simulink model "hdlcoder_ofdm_fft_eml_1024b"  (R2014a)
settings: Solver=FixedStepDiscrete  SolverMode=SingleTasking  StartTime=0.0  StopTime=35000  RelTol=1e-3
InitFcn:
  | wordLength = 16;
  | fracLength = 10;
  | TotalPoint= 1024;
  | TotalStage= 10;
  | FFT_nt=numerictype(1,12, 6);
  | twiddle_Signed = 1;
  | twiddle_WordLength = 12;
  | twiddle_FractionLength = 10;
  | twiddle_nt=numerictype(1,12, 10);
undefined symbols (not defined in the file): EbNodB, M
libraries: dspxfrm3 x3, commdigbbndpm3 x3, commsink2 x2, commchan3 x1, simulink x1, commrandsrc2 x1
Description:
  | OFDM Receiver with 512-Point Serial FFT
  | This model shows how to use Simulink(R) HDL Coder(TM) to check, generate,
  | and verify HDL code for a 512-point serial-FFT block built using the
  | MATLAB Function blocks and Simulink(R) blocks.
  | 
  | The 512-point serial-FFT block implements Radix-2 Dicimation-in-Time Cooley-Turkey algorithm.
  | It accepts streaming complex inputs and generate streaming complex outputs.
settings Model: DataTypeOverride=Double  FPTRunName=Active  Creator=mdonovan  LastModifiedBy=JohnE
settings DataIOCC: SaveOutput=off  SaveTime=off
settings OptimizationCC: BlockReduction=off  ConditionallyExecuteInputs=off  ExpressionDepthLimit=2147483647  InitFltsAndDblsToZero=on  EfficientMapNaN2IntZero=off
settings DebuggingCC: AlgebraicLoopMsg=error  UnderspecifiedInitializationDetection=Classic  MultiTaskDSMMsg=warning  MultiTaskCondExecSysMsg=none  SingleTaskRateTransMsg=error  IntegerOverflowMsg=none  FcnCallInpInsideContextMsg=UseLocalSettings  StateNameClashWarn=warning  LoggingUnavailableSignals=none
settings RTWCC: IncludeERTFirstTime=on
settings GRTTargetCC: CombineOutputUpdateFcns=off  GRTInterface=on

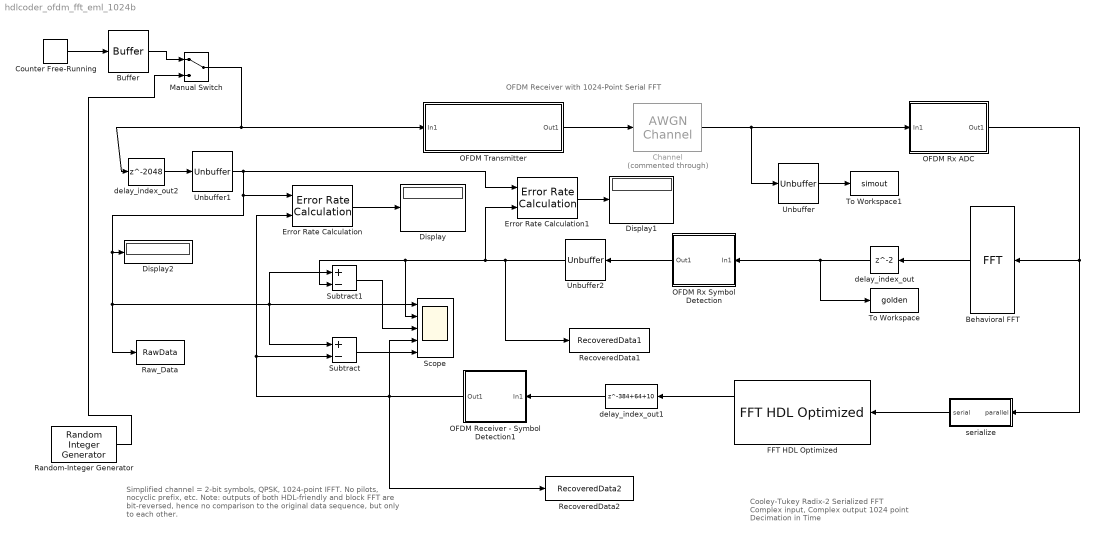
== system hdlcoder_ofdm_fft_eml_1024b ==
  note: Simplified channel = 2-bit symbols, QPSK, 1024-point IFFT.
      | No pilots, nocyclic prefix, etc.
      |
      | Note: outputs of both HDL-friendly and block FFT are bit-reversed,
      | hence no comparison to the original data sequence, but only to
      | each other.
  note: OFDM Receiver with 1024-Point Serial FFT
  note: Cooley-Tukey Radix-2 Serialized FFT
      | Complex input, Complex output
      | 1024 point
      | Decimation in Time
  Behavioral FFT : dspxfrm3/FFT  CompMethod=Table lookup  TableOpt=NEW  TableOptActive=Speed  BitRevOrder=on  InheritFFTLength=on  FFTLength=64  WrapInput=on  RowConvenienceOn=on  FFTImplementation=Auto  SkipNorm=off  firstCoeffMode=Specify word length  firstCoeffWordLength=11  firstCoeffFracLength=10  firstCoeffDataTypeStr=fixdt(1,11)  firstCoeffLastDataTypeStr=fixdt(1,11)  outputMode=Binary point scaling  outputWordLength=12  outputFracLength=6  outputDataTypeStr=fixdt(1,12,6)  outputLastDataTypeStr=fixdt(1,12,6)  outputMin=[]  outputMax=[]  accumMode=Binary point scaling  accumWordLength=25  accumFracLength=16  accumDataTypeStr=fixdt(1,25,16)  accumLastDataTypeStr=fixdt(1,25,16)  prodOutputMode=Binary point scaling  prodOutputWordLength=24  prodOutputFracLength=16  prodOutputDataTypeStr=fixdt(1,24,16)  prodOutputLastDataTypeStr=fixdt(1,24,16)  roundingMode=Floor  overflowMode=off
  Buffer : Buffer  N=1024  TreatMby1Signals=One channel
  Channel : commchan3/AWGN Channel  Commented=through  InputProcessing=Columns as channels (frame based)  seed=54321  noiseMode="Signal to noise ratio  (SNR)"  EbNodB=10  EsNodB=EbNodB+10*log10(log2(M))  SNRdB=100  bitsPerSym=1  Ps=1/1024  Tsym=Tsym  variance=10^(-0.1*15)/(2048*2)
  Counter Free-Running : simulink/Sources/Counter Free-Running  NumBits=2  tsamp=-1
  Display : Display
  Display1 : Display
  Display2 : Display
  Error Rate Calculation : commsink2/Error Rate Calculation  N=0  st_delay=1024  cp_mode=Entire frame  subframe=[]  PMode=Port  WsName=ErrorVec  RsMode2=off  stop=off  numErr=100  maxBits=1e6
  Error Rate Calculation1 : commsink2/Error Rate Calculation  N=0  st_delay=1024  cp_mode=Entire frame  subframe=[]  PMode=Port  WsName=ErrorVec  RsMode2=off  stop=off  numErr=100  maxBits=1e6
  FFT HDL Optimized : dspxfrm3/FFT HDL Optimized  SimulateUsing=Code generation  Normalize=off  FFTLengthSource=Property  FFTLength=1024  RoundingMethod=Nearest  OverflowAction=Saturate  ValidInputPort=off  StartOutputPort=off  EndOutputPort=off
  Manual Switch : ManualSwitch
  OFDM Receiver - Symbol Detection1 : Subsystem
  OFDM Rx ADC : Subsystem
  OFDM Rx Symbol Detection : Subsystem
  OFDM Transmitter : Subsystem
  Random-Integer Generator : commrandsrc2/Random Integer Generator  mul=4  seed=1234573  Ts=1  frameBased=on  sampPerFrame=1024  orient=off  outDataType=uint8
  Raw_Data : ToWorkspace  VariableName=RawData  SampleTime=-1
      settings: Save2DSignal=2-D array (concatenate along first dimension)
  RecoveredData1 : ToWorkspace  VariableName=RecoveredData1  SampleTime=-1
      settings: Save2DSignal=2-D array (concatenate along first dimension)
  "RecoveredData2 " : ToWorkspace  VariableName=RecoveredData2  SampleTime=-1
      settings: Save2DSignal=2-D array (concatenate along first dimension)
  Scope : Scope  NumInputPorts=5
      settings: YMin=-5~-5~-5~-5~-5  YMax=5~5~5~5~5  MaxDataPoints=50000
  Subtract : Sum  Inputs=+-
  Subtract1 : Sum  Inputs=+-  AccumDataTypeStr=fixdt(1,8,0)  OutDataTypeStr=Inherit: Same as accumulator
  To Workspace : ToWorkspace  VariableName=golden  SampleTime=-1
      settings: MaxDataPoints=1
  To Workspace1 : ToWorkspace  VariableName=simout  SampleTime=-1
      settings: Save2DSignal=2-D array (concatenate along first dimension)
  Unbuffer : Unbuffer  SampleBasedProcessing=Same as frame based
  Unbuffer1 : Unbuffer  SampleBasedProcessing=Same as frame based
  Unbuffer2 : Unbuffer  SampleBasedProcessing=Same as frame based
  delay_index_out : Delay  InputProcessing=Inherited  SampleTime=1024
  delay_index_out1 : Delay  DelayLength=384+64+10  InputProcessing=Inherited
  delay_index_out2 : Delay  DelayLength=2048  InputProcessing=Inherited  SampleTime=1024
  serialize : Subsystem
  wires:
  Channel/1 -> Unbuffer/1, OFDM Rx ADC/1(In1)
  OFDM Transmitter/1(Out1) -> Channel/1
  delay_index_out/1 -> OFDM Rx Symbol Detection/1(In1), To Workspace/1
  Behavioral FFT/1 -> delay_index_out/1
  Error Rate Calculation/1 -> Display/1
  serialize/1(serial) -> FFT HDL Optimized/1
  OFDM Rx ADC/1(Out1) -> serialize/1(parallel), Behavioral FFT/1
  OFDM Rx Symbol Detection/1(Out1) -> Unbuffer2/1
  OFDM Receiver - Symbol Detection1/1(Out1) -> Error Rate Calculation/2, Subtract/2, Scope/4, "RecoveredData2 "/1
  Manual Switch/1 -> delay_index_out2/1, OFDM Transmitter/1(In1)
  Unbuffer/1 -> To Workspace1/1
  Unbuffer1/1 -> Error Rate Calculation/1, Subtract1/1, Subtract/1, Scope/1, Raw_Data/1, Display2/1, Error Rate Calculation1/1
  FFT HDL Optimized/1 -> delay_index_out1/1
  delay_index_out1/1 -> OFDM Receiver - Symbol Detection1/1(In1)
  Subtract/1 -> Scope/5
  delay_index_out2/1 -> Unbuffer1/1
  Subtract1/1 -> Scope/3
  Unbuffer2/1 -> RecoveredData1/1, Error Rate Calculation1/2, Scope/2, Subtract1/2
  Error Rate Calculation1/1 -> Display1/1
  Counter Free-Running/1 -> Buffer/1
  Buffer/1 -> Manual Switch/1
  Random-Integer Generator/1 -> Manual Switch/2

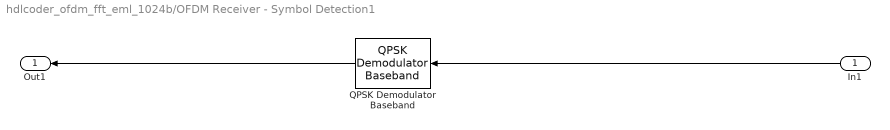
== system hdlcoder_ofdm_fft_eml_1024b/OFDM Receiver - Symbol Detection1 ==
  In1 : Inport
  QPSK Demodulator Baseband : commdigbbndpm3/QPSK Demodulator Baseband  Ph=pi/4  Dec=Gray  OutType=Integer  DecType=Hard decision  VarSource=Dialog  Variance=1  outDtype1=Inherit via internal rule  outDtype2=Inherit via internal rule  derotateFactorWordLen=16
  Out1 : Outport
  wires:
  QPSK Demodulator Baseband/1 -> Out1/1
  In1/1 -> QPSK Demodulator Baseband/1

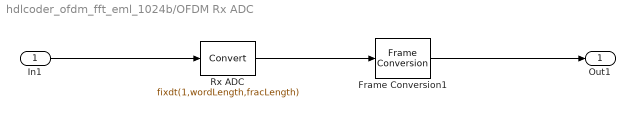
== system hdlcoder_ofdm_fft_eml_1024b/OFDM Rx ADC ==
  In1 : Inport
  Frame Conversion1 : FrameConversion  OutFrame=Sample-based
  Rx ADC : DataTypeConversion  OutDataTypeStr=fixdt(1,wordLength,fracLength)  SampleTime=1024
  Out1 : Outport
  wires:
  Rx ADC/1 -> Frame Conversion1/1
  Frame Conversion1/1 -> Out1/1
  In1/1 -> Rx ADC/1

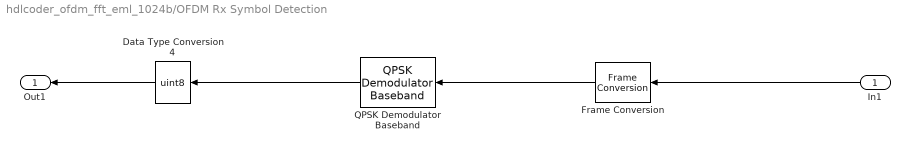
== system hdlcoder_ofdm_fft_eml_1024b/OFDM Rx Symbol Detection ==
  In1 : Inport
  Data Type Conversion4 : DataTypeConversion  OutDataTypeStr=uint8
  Frame Conversion : FrameConversion
  QPSK Demodulator Baseband : commdigbbndpm3/QPSK Demodulator Baseband  Ph=pi/4  Dec=Gray  OutType=Integer  DecType=Hard decision  VarSource=Dialog  Variance=1  outDtype1=Inherit via internal rule  outDtype2=Inherit via internal rule  derotateFactorWordLen=16
  Out1 : Outport
  wires:
  QPSK Demodulator Baseband/1 -> Data Type Conversion4/1
  In1/1 -> Frame Conversion/1
  Frame Conversion/1 -> QPSK Demodulator Baseband/1
  Data Type Conversion4/1 -> Out1/1

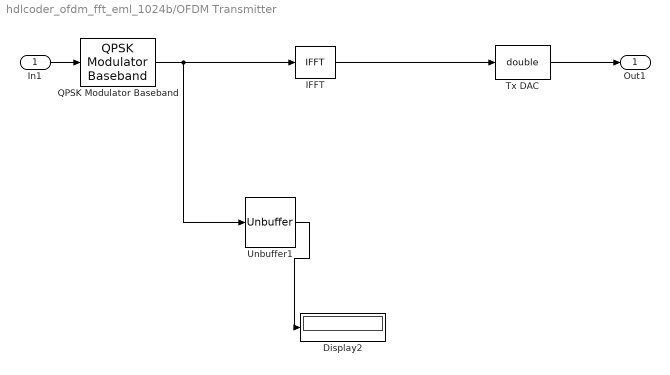
== system hdlcoder_ofdm_fft_eml_1024b/OFDM Transmitter ==
  In1 : Inport
  Display2 : Display
  IFFT : dspxfrm3/IFFT  CompMethod=Table lookup  TableOpt=HYBRID  TableOptActive=Speed  BitRevOrder=on  cs_in=off  SkipNorm=on  InheritFFTLength=on  FFTLength=64  WrapInput=on  mode=Complex  outSamplingMode=Frame based  RowConvenienceOn=on  FFTImplementation=Auto  firstCoeffMode=Specify word length  firstCoeffWordLength=16  firstCoeffFracLength=15  firstCoeffDataTypeStr=fixdt(1,16)  firstCoeffLastDataTypeStr=fixdt(1,16)  outputMin=[]  outputMax=[]  accumDataTypeStr=Inherit: Same as product output  accumLastDataTypeStr=Inherit: Same as product output  roundingMode=Floor  overflowMode=off
  QPSK Modulator Baseband : commdigbbndpm3/QPSK Modulator Baseband  InType=Integer  Enc=Gray  Ph=pi/4  outDtype=Fixed-point  outWordLen=12  outUDDataType=sfix(16)  outFracLenMode=User-defined  outFracLen=6
  Tx DAC : DataTypeConversion  OutDataTypeStr=double
  Unbuffer1 : Unbuffer  SampleBasedProcessing=Same as frame based
  Out1 : Outport
  wires:
  QPSK Modulator Baseband/1 -> IFFT/1, Unbuffer1/1
  IFFT/1 -> Tx DAC/1
  In1/1 -> QPSK Modulator Baseband/1
  Tx DAC/1 -> Out1/1
  Unbuffer1/1 -> Display2/1

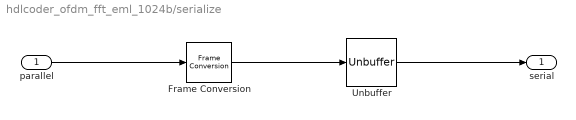
== system hdlcoder_ofdm_fft_eml_1024b/serialize ==
  parallel : Inport
  Frame Conversion : FrameConversion
  Unbuffer : Unbuffer  SampleBasedProcessing=Same as frame based
  serial : Outport
  wires:
  parallel/1 -> Frame Conversion/1
  Frame Conversion/1 -> Unbuffer/1
  Unbuffer/1 -> serial/1
